simulink model "vehicle_model_controller"  (R2020b)
settings: Solver=VariableStepAuto  StartTime=0.0  StopTime=10.0  RelTol=1e-3
undefined symbols (not defined in the file or in its folder): BWLF, BWRF, front_forces, FWLF, FWRF, rear_forces
libraries: nesl_utility x24, sdl_lib x16, fl_lib x4, autolibmappedmotor x4, autolibdatasheetbattery x1, vehdynlibsteering x1, pid_lib x1, autolibshared x1
(part 2 of 2)

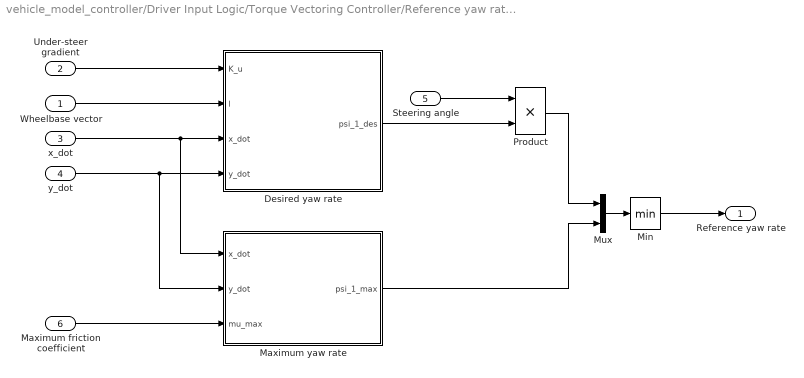
== system vehicle_model_controller/Driver Input Logic/Torque Vectoring Controller/Reference yaw rate processor ==
  Wheelbase vector : Inport
  Under-steer gradient : Inport  Port=2
  x_dot : Inport  Port=3
  y_dot : Inport  Port=4
  "Steering angle " : Inport  Port=5
  Maximum friction coefficient : Inport  Port=6
  Desired yaw rate : MATLAB Function  TreatAsAtomicUnit=on
  Maximum yaw rate : MATLAB Function  TreatAsAtomicUnit=on
  Min : MinMax
  Mux : Mux  Inputs=2
  Product : Product
  Reference yaw rate : Outport
  wires:
  Wheelbase vector/1 -> Desired yaw rate/2(l)
  Under-steer gradient/1 -> Desired yaw rate/1(K_u)
  Desired yaw rate/1(psi_1_des) -> Product/2
  Min/1 -> Reference yaw rate/1
  Maximum friction coefficient/1 -> Maximum yaw rate/3(mu_max)
  "Steering angle "/1 -> Product/1
  y_dot/1 -> Maximum yaw rate/2(y_dot), Desired yaw rate/4(y_dot)
  x_dot/1 -> Maximum yaw rate/1(x_dot), Desired yaw rate/3(x_dot)
  Mux/1 -> Min/1
  Product/1 -> Mux/1
  Maximum yaw rate/1(psi_1_max) -> Mux/2

== matlab function vehicle_model_controller/Driver Input Logic/Torque Vectoring Controller/Yaw rate error ==
  data: psi_1 input; psi_1_error output; psi_1_ref input
function psi_1_error = yaw_rate_error(psi_1, psi_1_ref)
%% Yaw rate error
% Developers:    David Farell
%                Elliot Stockwell
% Developed for: Purdue Electric Racing
% Date:          08/31/2021
%
% Definitions:
% psi_1_ref:  reference yaw rate                    [rad * s^-1]
% psi_1:    yaw rate                                [rad * s^-1]

%% Calculating yaw rate error
psi_1_error = psi_1_ref - psi_1;
% Calculates the yaw rate error for the PID controller to operate on

== matlab function vehicle_model_controller/Driver Input Logic/Torque Vectoring Controller/LP model ==
  data: s input; T_x_ij output; l input; PID input; delta input; F_x_ij_max input; driver_input input
function T_x_ij = LP(s, l, PID, delta, F_x_ij_max, driver_input)
%% Two-track model equation of motion
% Developers:    David Farell
%                Elliot Stockwell
% Developed for: Purdue Electric Racing
% Date:          04/24/2021
%
% Definitions:
% s:        half track width vector                 [m]
% l:        wheelbase vector                        [m]
% delta:    steering angle vector                   [deg]
% PID:      efficacy of LP based on error           [N]
% F_x_ij_max:   maximum longitudinal tire force vector          [N]
% driver_input: maximum total force motors can output           [N]

%% Constants
J_z = 1;        % Inertia moment                            [kg * m^2]
s_f = s(1);     % half track width front                    [m]
s_r = s(2);     % half track width rear                     [m]
l_f = l(1);     % wheelbase front                           [m]
l_r = l(2);     % wheelbase rear                            [m]
% F_y_fl = F_y_ij(1); % lateral tire force (front left tire)  [N]
% F_y_fr = F_y_ij(2); % lateral tire force (front right tire) [N]
% F_y_rl = F_y_ij(3); % lateral tire force (rear left tire)   [N]
% F_y_rr = F_y_ij(4); % lateral tire force (rear right tire)  [N]
LB = 0;         % wheel force lower bound                   [N]
UP = 100;       % wheel force upper bound                   [N]
R = 0.3;        % wheel radius                              [m]

%% Defining EOM vector K_1
% x_1 component of EOM vector in K_1
x_1 = (-s_f * cos(delta)) + (l_f * sin(delta));    
% x_2 component of EOM vector in K_1
x_2 = (s_f * cos(delta)) + (l_f * sin(delta));     
% x_3 component of EOM vector in K_1
x_3 = -s_r;     
% x_4 component of EOM vector in K_1
x_4 = s_r; 
% EOM vector in K_1
x = [x_1; x_2; x_3; x_4]; 

% K_1 vector of vehicle constants and parameters
K_1 = (1 / J_z) * x; 

%% Defining EOM linear combination K_2
% y_1 component of EOM linear combination in K_2
y_1 = (s_f * sin(delta)) + (l_f * cos(delta));    
% y_2 component of EOM linear combination in K_2
y_2 = (-s_f * sin(delta)) + (l_f * cos(delta));
% y_3 component of EOM linear combination in K_2
y_3 = -l_r;
% y_4 component of EOM vector in K_2
y_4 = -l_r;
% EOM vector in K_2
y = [y_1; y_2; y_3; y_4]; 

% K_2 vector of vehicle constants and parameters and lateral wheel forces
K_2 = (1 / J_z) * y;


%% Linear Programming Model
% The solution output of the linear programming model is a variable
% F_x_ij_mod, which is equal to the requested linear force plus a slack
% variable (maximum linear motor output) to ensure the solution is positive

% Define constraints

F_x_ij_mod = optimvar('F_x_ij','LowerBound',LB,'UpperBound',UP);

% Linear programming constants
F_sv = [100; 100; 100; 100];    % slack variable      [N]
% The slack variable ensures the optimization statement is always positive
% through the solving process and is set to the maximum possible linear 
% output of each motor; it is subtracted from the solution at the end


% Create optimization
linprob = optimproblem('Objective',F_x_ij_max - F_x_ij_mod + F_sv + err);
% Minimizes the objective function [Maximum longitudinal force] - 
% [Adjusted requested longitudinal force] + [slack variable to keep 
% solution positive] + [exact penalty function constraining solution to 
% wheel traction limit]

% Define linear constriants (inequalities)
% Below two constriants define the bounds of F_x_ij_mod, as it cannot be
% larger than the maximum possible linear force plus the slack variable nor
% can it be smaller than the maximum negative possible linear force plus
% the slack variable
linprob.Constraints.cons1 = F_sv + F_x_ij_max >= F_x_ij_mod;
% The adjusted requested linear force F_x_ij_mod must be less than or
% equal to the slack variable F_sv plus the maximum possible linear force 
% at each motor F_x_ij_max (rearranging gives [max linear force] >= 
% [unadjusted requested linear force])
linprob.Constraints.cons2 = F_sv - F_x_ij_max <= F_x_ij_mod;
% The adjusted requested linear force F_x_ij_mod must be greater than or 
% equal to the slack variable F_sv minus the maximum possible linear force
% at each motor F_x_ij_max (rearranging gives -[max linear force] <=
% [unadjusted requested linear force])
linprob.Constraints.cons3 = F_tot + 4 * F_sv >= sum(F_x_ij_mod);
% The adjusted requested linear force F_x_ij_mod must be less than or equal
% to the total demanded torque F_tot plus four times the slack variable
% F_sv (rearranging gives [Total demanded linear force] >= [unadjusted
% requested linear force])

% Define linear constraints (equalities)
linprob.Constraints.econs1 = err == exp(1000 .* (F_x_ij - F_x_ij_max)).';
% Impose massive error term as soon as the optimization model lands on a 
% solution greater than the maximum possible requested linear force - THIS
% NEEDS TO BE REPLACED BY AN APPROXIMATION OF THE TRACTION CIRCLE SET EQUAL
% TO THE EXACT PENALTY FUNCTION
linprob.Constraints.econs1 = K_1 .* f_x_ij_mod == -K_2 + PID + ...
    K_1 .* F_sv + err;
% The vehicle parameters and constants at all four wheels K_1 multiplied by
% the adjusted requested linear force at each wheel F_x_ij_mod must be
% equal to the negative of the vehicle parameters, constants and forces at 
% each wheel K_2 plus the proportional and integral error of the yaw rate
% PID plus the vehicle parameters and constants at all four wheels K_1
% multiplied by the slack variable F_sv plus the exact penalty function err

% Solve problem
linsol = solve(linprob);

% Adjust with slack variable
F_x_ij = linsol - F_sv;
% Removes the slack variable F_sv that was keeping the solution positive 
% during the solving process from F_x_ij_mod 

% Convert to required torque
T_x_ij = F_x_ij .* R;

== matlab function vehicle_model_controller/Driver Input Logic/Torque Vectoring Controller/Reference yaw rate processor/Desired yaw rate ==
  data: K_u input; l input; x_dot input; y_dot input; psi_1_des output
function psi_1_des = des_yaw_rate(K_u, l, x_dot, y_dot)
%% Desired yaw rate
% Developers:    David Farell
%                Elliot Stockwell
% Developed for: Purdue Electric Racing
% Date:          04/24/2021
%
% Definitions:
% x_dot:    longitudinal velocity at CoG            [m * s^-1]
% y_dot:    lateral velocity at CoG                 [m * s^-1]
% l:        wheelbase vector                        [m]
% K_u:      under-steer gradient                    [unitless]
% delta:    steering angle                          [deg]

%% Constants
v_cog = sqrt(x_dot^2 + y_dot^2); % speed at CoG            [m * s^-1]
l_f = l(1);      % wheelbase front                         [m]
l_r = l(2);      % wheelbase rear                          [m]

%% Desired yaw rate
psi_1_des = v_cog / ((l_f + l_r) + (K_u * v_cog ^ 2));
% calculates desired yaw rate based on the equations given in the TV paper
% by Anton Stoop

== matlab function vehicle_model_controller/Driver Input Logic/Torque Vectoring Controller/Reference yaw rate processor/Maximum yaw rate ==
  data: x_dot input; y_dot input; psi_1_max output; mu_max input
function psi_1_max = max_yaw_rate(x_dot, y_dot, mu_max)
%% Maximum yaw rate
% Developers:    David Farell
%                Elliot Stockwell
% Developed for: Purdue Electric Racing
% Date:          04/24/2021
%
% Definitions:
% x_dot:    longitudinal velocity at CoG            [m * s^-1]
% y_dot:    lateral velocity at CoG                 [m * s^-1]
% mu_max:   maximum friction coefficient            [unitless]

%% Constants
g = 9.806;       % acceleration due to gravity             [m / s^-2]

%% Calculations
v_cog = sqrt(x_dot^2 + y_dot^2); % speed at CoG            [m * s^-1]
mu_max = max(max(mu_max)); % maximum overall friction coefficient 

%% Maximum yaw rate
psi_1_max = (mu_max * g) / (v_cog + 0.05);

== matlab function vehicle_model_controller/Driver Input Logic/Torque Vectoring Controller/Maximum longitudinal force, no slip ==
  data: mu_max input; delta input; alpha input; F_x_ij input; F_z_ij input; F_x_ij_max output
function F_x_ij_max = LP_F_x_max_noslip(mu_max, delta, alpha, ...
      F_x_ij, F_z_ij)
%% Linear programming max longitudinal force before loss of traction
% Developers:    David Farell
%                Elliot Stockwell
% Developed for: Purdue Electric Racing
% Date:          04/24/2021
%
% Definitions:
% F_x_ij:   Tire lateral force vector               [N]
% F_z_ij:   Tire loading vector                     [N]
% mu_max:   Maximum friction coefficient            [m/s]
% alpha:    Slip angle vector                       [rad]
% delta:    Steering angle                          [rad]
% req_f:    Driver requested force                  [N]

%% Constants
delta_o = [delta(1); delta(2); 0; 0];
mu_max = [mu_max(1:2), mu_max(3:4)]';

%% Maximum longitudinal forces in the direction of wheel velocity
F_wl = sqrt((mu_max .* F_z_ij).^2 + F_x_ij.^2);

%% Maximum longitudinal and lateral forces in the wheel coordinates
F_l = F_wl .* cos(alpha) + F_x_ij .* sin(alpha);
F_s = F_x_ij .* cos(alpha) - F_wl .* sin(alpha);

% Maximum longitudinal forces in undercarriage coordinates
F_x_ij_max = F_l .* cos(delta_o) - F_s .* sin(delta_o);

== matlab function vehicle_model_controller/Driver Input Logic/Torque Vectoring Controller/MATLAB Function ==
  data: delta input; y_dot input; x_dot input; r input; w input; alpha output; s input
function alpha = slip_angle(delta, y_dot, x_dot, r, w, s)
%% Front and rear slip angle
% Developers:    David Farell
%                Elliot Stockwell
% Developed for: Purdue Electric Racing
% Date:          04/27/2021
%
% Definitions:
% y_dot:    Vehicle CoG lateral velocity            [m/s]
% x_dot:    Vehicle CoG longitudinal velocity       [m/s]    
% a:        Distance from front wheel axle to CoG   [m]
% b:        Distance from rear wheel axle to CoG    [m]
% r:        Vehicle angular velocity                [rad/s]
% w:        Wheelbase vector                        [m]
% delta:    Steering angle vector                   [rad]

%% Constants
a = s(1);
b = s(2);
w_f = w(1);
w_r = w(2);
delta_fl = delta(1);
delta_fr = delta(2);
delta_rl = 0;
delta_rr = 0;

%% Front left slip angle
alpha_fl = atan((y_dot + a * r) / (x_dot + r * w_f / 2)) - delta_fl;

%% Front right slip angle
alpha_fr = atan((y_dot + a * r) / (x_dot - r * w_f / 2)) - delta_fr;

%% Rear left slip angle
alpha_rl = atan((y_dot - b * r) / (x_dot + r * w_r / 2)) - delta_rl;

%% Rear right slip angle
alpha_rr = atan((y_dot - b * r) / (x_dot - r * w_r / 2)) - delta_rr;


%% Slip angle vector
alpha = [alpha_fl; alpha_fr; alpha_rl; alpha_rr];

== matlab function vehicle_model_controller/Electric Vehicle Body/Mechanical Braking Effects/mechanical_braking_effects ==
  data: braking_forces input; front_forces input; FwF output; rear_forces input; FwR output
function [FwF, FwR] = Mechanical_Braking_Effects(braking_forces, front_forces, rear_forces)
%% Mechanical Braking Effects
% Developers:    Demetrius Gulewicz
% Developed for: Purdue Electric Racing
% Date:          09/01/2021
%
% Definitions:
% front_force:      force vector from the front motors    [N]
% braking_forces:   braking force vector on all 4 tires   [N]
% rear_forces:      force vector from the rear motors     [N]

%% Calculation
FwF = front_forces' - braking_forces(1:2);
FwR = rear_forces' - braking_forces(3:4);

== matlab function vehicle_model_controller/Driver Input Logic/Braking Controller/MATLAB Function ==
  data: driver_input input; T_x_ij output
function T_x_ij = split_braking_torque(driver_input)
%% Regenerative Braking Force Split
% Developers:    Demetrius Gulewicz
% Developed for: Purdue Electric Racing
% Date:          09/01/2021
%
% Definitions:
% driver_input:   sum of forces requested by driver to the 4 motors   [N]
%% Constants
R = 0.3;        % wheel radius                              [m]


%% Calculation
driver_torque = (driver_input * R)/ 4;


T_x_ij = [driver_torque; driver_torque; driver_torque; driver_torque];
